simulink library "vhcl2turbLinearize_cl"  (R2020a)
settings: Solver=VariableStepAuto  StartTime=0.0  StopTime=10.0  RelTol=1e-3
undefined symbols (not defined in the file): env, VEHICLE, vhcl
libraries: vrlib x2, addedMass_cl x1, Copy_of_fluidDynamicSurface_cl x1, alphaBeta_ul x1, dragTurbineMantaNew_ul x1, fuselage_cl x1, sixDoFDynamics_cl x1, tethersMoment_cl x1, thrAttachPtKinematics_ul x1
settings Model: Creator=mcobb  LastModifiedBy=andre
settings DataIOCC: ReturnWorkspaceOutputs=off
settings DebuggingCC: ArithmeticOperatorsInVariantConditions=warning
settings SFSimCC: CustomCodeUndefinedFunction=UseInterfaceOnly

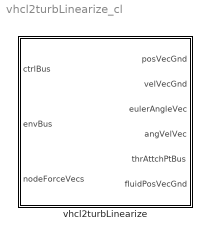
== system vhcl2turbLinearize_cl ==
  vhcl2turbLinearize : Subsystem  VariantControl=strcmpi(VEHICLE,'vehicleManta2Rot')  mask{vcl=vhcl, rho=env.water.density.Value, grav=env.gravAccel.Value}
      mask prompts: vcl "Vehicle"; rho "Density"; grav "Gravity"
      mask DialogControl Container9 Prompt: General
      mask DialogControl Container5 Prompt: Vehicle object (OCT.vehicle)
      mask DialogControl ParameterGroupVar Prompt: Environment Object (OCT.env)
      mask Display:
      | image('kite2.PNG',[0 0 700 700]/4,'on')
      | 
      | port_label('input',1,'ctrlBus')
      | port_label('input',2,'envBus')
      | port_label('input',3,'nodeForceVecs')
      | 
      | port_label('output',1,'posVecGnd')
      | port_label('output',2,'velVecGnd')
      | port_label('output',3,'eulAng')
      | port_label('output',4,'angVelVec')
      | port_label('output',5,'thrAttchPtBus')
      | port_label('output',6,'fluidPosVecGnd')

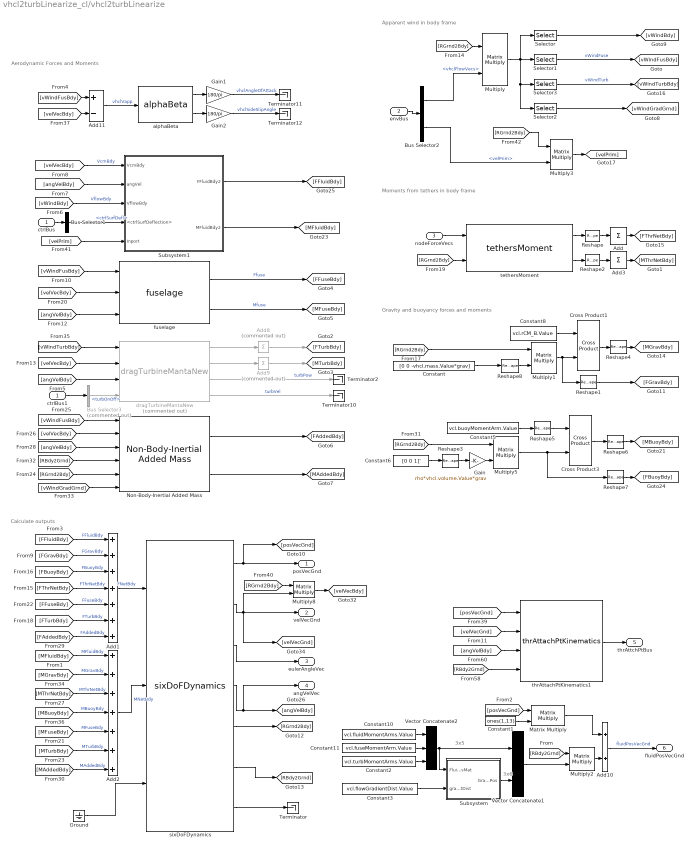
== system vhcl2turbLinearize_cl/vhcl2turbLinearize ==
  note: 3x6
  note: 3x5
  note: Calculate outputs
  note: Apparent wind in body frame
  note: Gravity and buoyancy forces and moments
  note: Moments from tethers in body frame
  note: Aerodynamic Forces and Moments
  ctrlBus : Inport  OutDataTypeStr=Bus: fltCtrlBus
  envBus : Inport  Port=2  OutDataTypeStr=Bus: envBus
  nodeForceVecs : Inport  Port=3
  Add : Sum  Inputs=+  CollapseMode=Specified dimension  CollapseDim=2
  Add1 : Sum  Inputs=+++++++
  Add10 : Sum
  Add11 : Sum  Inputs=+-
  Add2 : Sum  Inputs=+++++++
  Add3 : Sum  Inputs=+  CollapseMode=Specified dimension  CollapseDim=2
  Add8 : Sum  Commented=on  Inputs=1  CollapseMode=Specified dimension  CollapseDim=2
  Add9 : Sum  Commented=on  Inputs=1  CollapseMode=Specified dimension  CollapseDim=2
  Bus Selector1 : BusSelector  OutputSignals=ctrlSurfDefl
  Bus Selector2 : BusSelector  OutputSignals=vhclFlowVecs,velPrim
  Bus Selector3 : BusSelector  Commented=on  OutputSignals=turbOnOff
  Constant : Constant  Value=[0 0 -vhcl.mass.Value*grav]
  Constant1 : Constant  Value=ones(1,13)  VectorParams1D=off
  Constant10 : Constant  Value=vcl.fluidMomentArms.Value
  Constant11 : Constant  Value=vcl.fuseMomentArm.Value
  Constant2 : Constant  Value=vcl.turbMomentArms.Value
  Constant3 : Constant  Value=vcl.flowGradientDist.Value
  Constant5 : Constant  Value=vcl.buoyMomentArm.Value
  Constant6 : Constant  Value=[0 0 1]'
  Constant8 : Constant  Value=vcl.rCM_B.Value
  Cross Product1 : vrlib/Utilities/Cross Product
  Cross Product3 : vrlib/Utilities/Cross Product
  Gain : Gain  Gain=rho*vhcl.volume.Value*grav
  Gain1 : Gain  Gain=180/pi
  Gain2 : Gain  Gain=180/pi
  Ground : Ground
  Matrix Multiply : Product  Multiplication=Matrix(*)
  Multiply{,1..3,5,8} (6 alike) : Product  Multiplication=Matrix(*)
  Non-Body-Inertial Added Mass : addedMass_cl/Non-Body-Inertial Added Mass  MaMat=vcl.Ma6x6_LE.Value  rB_LE=vcl.rB_LE.Value  gradDist=vcl.flowGradientDist.Value
  Reshape : Reshape  OutputDimensionality=Customize  OutputDimensions=[3 vcl.numTethers.Value]
  Reshape{1,3..8} (7 alike) : Reshape  OutputDimensionality=Column vector (2-D)
  Reshape2 : Reshape  OutputDimensionality=Customize  OutputDimensions=[3 vcl.numTethers.Value]
  Selector : Selector  NumberOfDimensions=2  InputPortWidth=3  IndexOptions=Select all,Index vector (dialog)  Indices=[1 3],1:4  OutputSizes=1,1
  Selector1 : Selector  NumberOfDimensions=2  InputPortWidth=3  IndexOptions=Select all,Index vector (dialog)  Indices=[1 3],5  OutputSizes=1,1
  Selector2 : Selector  NumberOfDimensions=2  InputPortWidth=3  IndexOptions=Select all,Index vector (dialog)  Indices=[1 3],8:13  OutputSizes=1,1
  Selector3 : Selector  NumberOfDimensions=2  InputPortWidth=3  IndexOptions=Select all,Index vector (dialog)  Indices=[1 3],6:7  OutputSizes=1,1
  Subsystem : Subsystem
  Subsystem1 : Subsystem
  Terminator{,2,10..12} (5 alike) : Terminator
  Vector Concatenate1 : Concatenate  Mode=Multidimensional array  ConcatenateDimension=2
  Vector Concatenate2 : Concatenate  NumInputs=3  Mode=Multidimensional array  ConcatenateDimension=2
  alphaBeta : alphaBeta_ul/alphaBeta  SystemSampleTime=-1  Latency=0  AutoFrameSizeCalculation=off
  ctrlBus1 : InportShadow  OutDataTypeStr=Bus: fltCtrlBus
  dragTurbineMantaNew : dragTurbineMantaNew_ul/dragTurbineMantaNew  Commented=on  rho_fluid=rho  turb_struct=vcl.struct('OCT.turb')
  fuselage : fuselage_cl/fuselage  momArm=vcl.fuseMomentArm.Value  fus=vcl.fuse  fusRhoDa=rho
  sixDoFDynamics : sixDoFDynamics_cl/sixDoFDynamics  vcl=vcl
      link override sixDoFDynamicsCoupledCM: MMat=vcl.M6x6_B.Value  MaMat=vcl.Ma6x6_LE.Value  rB_LE=vcl.rB_LE.Value
  tethersMoment : tethersMoment_cl/tethersMoment  arms=vcl.struct('OCT.thrAttch')
  thrAttachPtKinematics1 : thrAttachPtKinematics_ul/thrAttachPtKinematics  atchPts=vcl.struct('OCT.thrAttch')
  posVecGnd : Outport  VectorParamsAs1DForOutWhenUnconnected=off
  velVecGnd : Outport  Port=2  VectorParamsAs1DForOutWhenUnconnected=off
  eulerAngleVec : Outport  Port=3  VectorParamsAs1DForOutWhenUnconnected=off
  angVelVec : Outport  Port=4  VectorParamsAs1DForOutWhenUnconnected=off
  thrAttchPtBus : Outport  Port=5  VectorParamsAs1DForOutWhenUnconnected=off
  fluidPosVecGnd : Outport  Port=6  VectorParamsAs1DForOutWhenUnconnected=off
  wires:
  sixDoFDynamics/3 -> eulerAngleVec/1
  sixDoFDynamics/1 -> [posVecGnd], posVecGnd/1
  sixDoFDynamics/2 -> Multiply8/2, [velVecGnd], velVecGnd/1
  thrAttachPtKinematics1/1 -> thrAttchPtBus/1
  ctrlBus/1 -> Bus Selector1/1
  [vWindFusBdy] -> fuselage/1
  [velVecBdy] -> fuselage/2
  [angVelBdy] -> fuselage/3
  [vWindTurbBdy] -> dragTurbineMantaNew/1
  [velVecBdy] -> dragTurbineMantaNew/2
  [angVelBdy] -> dragTurbineMantaNew/3
  dragTurbineMantaNew/1 -> Add8/1
  dragTurbineMantaNew/2 -> Add9/1
  Add8/1 -> [FTurbBdy]
  Add9/1 -> [MTurbBdy]
  dragTurbineMantaNew/3 -> Terminator2/1  "turbPow"
  [vWindFusBdy] -> Non-Body-Inertial Added Mass/1
  [velVecBdy] -> Non-Body-Inertial Added Mass/2
  [angVelBdy] -> Non-Body-Inertial Added Mass/3
  [RBdy2Grnd] -> Non-Body-Inertial Added Mass/4
  [RGrnd2Bdy] -> Non-Body-Inertial Added Mass/5
  [vWindGradGrnd] -> Non-Body-Inertial Added Mass/6
  Constant6/1 -> Reshape3/1
  Reshape3/1 -> Gain/1
  [RGrnd2Bdy] -> Multiply5/1
  Gain/1 -> Multiply5/2
  Constant5/1 -> Reshape5/1
  Reshape5/1 -> Cross Product3/1
  Cross Product3/1 -> Reshape6/1
  Reshape6/1 -> [MBuoyBdy]
  Multiply5/1 -> Reshape7/1, Cross Product3/2
  Reshape7/1 -> [FBuoyBdy]
  Reshape1/1 -> [FGravBdy]
  Multiply1/1 -> Reshape1/1, Cross Product1/2
  fuselage/1 -> [FFuseBdy]  "Ffuse"
  fuselage/2 -> [MFuseBdy]  "Mfuse"
  Constant/1 -> Reshape8/1
  [RGrnd2Bdy] -> Multiply1/1
  Reshape8/1 -> Multiply1/2
  Constant8/1 -> Cross Product1/1
  Cross Product1/1 -> Reshape4/1
  Reshape4/1 -> [MGravBdy]
  [RGrnd2Bdy] -> tethersMoment/2
  nodeForceVecs/1 -> tethersMoment/1
  tethersMoment/1 -> Reshape/1
  tethersMoment/2 -> Reshape2/1
  Reshape/1 -> Add/1
  Reshape2/1 -> Add3/1
  Add/1 -> [FThrNetBdy]
  Add3/1 -> [MThrNetBdy]
  [RGrnd2Bdy] -> Multiply/1
  envBus/1 -> Bus Selector2/1
  Bus Selector2/1 -> Multiply/2  "<vhclFlowVecs>"
  Multiply/1 -> Selector/1, Selector2/1, Selector3/1, Selector1/1
  Selector/1 -> [vWindBdy]
  Selector1/1 -> [vWindFusBdy]  "vWindFuse"
  Selector2/1 -> [vWindGradGrnd]
  [RGrnd2Bdy] -> Multiply8/1
  Multiply8/1 -> [velVecBdy]
  [FFluidBdy] -> Add1/1  "FFluidBdy"
  [FGravBdy] -> Add1/2  "FGravBdy"
  [FBuoyBdy] -> Add1/3  "FBuoyBdy"
  [FThrNetBdy] -> Add1/4  "FThrNetBdy"
  [FFuseBdy] -> Add1/5  "FFuseBdy"
  [FTurbBdy] -> Add1/6  "FTurbBdy"
  [FAddedBdy] -> Add1/7  "FAddedBdy"
  Add1/1 -> sixDoFDynamics/1  "FNetBdy"
  [MFluidBdy] -> Add2/1  "MFluidBdy"
  [MGravBdy] -> Add2/2  "MGravBdy"
  [MThrNetBdy] -> Add2/3  "MThrNetBdy"
  [MBuoyBdy] -> Add2/4  "MBuoyBdy"
  [MFuseBdy] -> Add2/5  "MFuseBdy"
  [MTurbBdy] -> Add2/6  "MTurbBdy"
  [MAddedBdy] -> Add2/7  "MAddedBdy"
  Add2/1 -> sixDoFDynamics/2  "MNetBdy"
  sixDoFDynamics/5 -> [RGrnd2Bdy]
  sixDoFDynamics/6 -> [RBdy2Grnd]
  [posVecGnd] -> thrAttachPtKinematics1/1
  [velVecGnd] -> thrAttachPtKinematics1/2
  [angVelBdy] -> thrAttachPtKinematics1/3
  [RBdy2Grnd] -> thrAttachPtKinematics1/4
  Constant10/1 -> Vector Concatenate2/1
  Constant11/1 -> Vector Concatenate2/2
  Vector Concatenate2/1 -> Vector Concatenate1/1, Subsystem/1(FluidCentPosMat)
  Constant3/1 -> Subsystem/2(gradientDist)
  Subsystem/1(GradientFlowPos) -> Vector Concatenate1/2
  sixDoFDynamics/4 -> [angVelBdy], angVelVec/1
  Vector Concatenate1/1 -> Multiply2/2
  [RBdy2Grnd] -> Multiply2/1
  Multiply2/1 -> Add10/2
  Matrix Multiply/1 -> Add10/1
  Add10/1 -> fluidPosVecGnd/1  "fluidPosVecGnd"
  Constant1/1 -> Matrix Multiply/2
  [posVecGnd] -> Matrix Multiply/1
  Bus Selector3/1 -> dragTurbineMantaNew/4  "<turbOnOff>"
  ctrlBus1/1 -> Bus Selector3/1
  Constant2/1 -> Vector Concatenate2/3
  Selector3/1 -> [vWindTurbBdy]  "vWindTurb"
  dragTurbineMantaNew/4 -> Terminator10/1  "turbVel"
  Non-Body-Inertial Added Mass/1 -> [FAddedBdy]
  Non-Body-Inertial Added Mass/2 -> [MAddedBdy]
  [vWindFusBdy] -> Add11/1
  Add11/1 -> alphaBeta/1  "vhclVapp"
  [velVecBdy] -> Add11/2
  alphaBeta/2 -> Gain2/1
  Gain1/1 -> Terminator11/1  "vhclAngleOfAttack"
  alphaBeta/1 -> Gain1/1
  Gain2/1 -> Terminator12/1  "vhclSideSlipAngle"
  [velVecBdy] -> Subsystem1/1(VcmBdy)  "VcmBdy"
  [angVelBdy] -> Subsystem1/2(angVel)
  [vWindBdy] -> Subsystem1/3(VflowBdy)  "VflowBdy"
  Bus Selector1/1 -> Subsystem1/4(<ctrlSurfDeflection>)  "<ctrlSurfDefl>"
  Subsystem1/1(FFluidBdy2) -> [FFluidBdy]
  Subsystem1/2(MFluidBdy2) -> [MFluidBdy]
  Bus Selector2/2 -> Multiply3/2  "<velPrim>"
  [velPrim] -> Subsystem1/5(Inport)
  [RGrnd2Bdy] -> Multiply3/1
  Multiply3/1 -> [velPrim]
  Ground/1 -> sixDoFDynamics/3
  sixDoFDynamics/7 -> Terminator/1

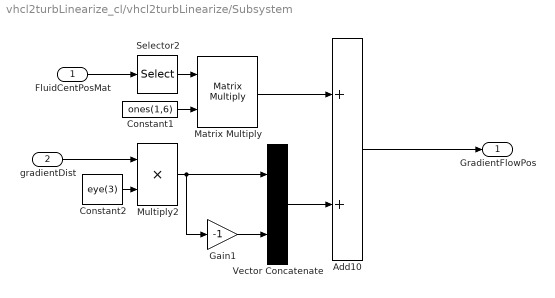
== system vhcl2turbLinearize_cl/vhcl2turbLinearize/Subsystem ==
  FluidCentPosMat : Inport
  gradientDist : Inport  Port=2
  Add10 : Sum
  Constant1 : Constant  Value=ones(1,6)  VectorParams1D=off
  Constant2 : Constant  Value=eye(3)
  Gain1 : Gain  Gain=-1
  Matrix Multiply : Product  Multiplication=Matrix(*)
  Multiply2 : Product
  Selector2 : Selector  NumberOfDimensions=2  InputPortWidth=3  IndexOptions=Select all,Index vector (dialog)  Indices=[1 3],5  OutputSizes=1,1
  Vector Concatenate : Concatenate  Mode=Multidimensional array  ConcatenateDimension=2
  GradientFlowPos : Outport  VectorParamsAs1DForOutWhenUnconnected=off
  wires:
  FluidCentPosMat/1 -> Selector2/1
  Vector Concatenate/1 -> Add10/2
  Selector2/1 -> Matrix Multiply/1
  Multiply2/1 -> Gain1/1, Vector Concatenate/1
  Constant1/1 -> Matrix Multiply/2
  Matrix Multiply/1 -> Add10/1
  Gain1/1 -> Vector Concatenate/2
  Constant2/1 -> Multiply2/2
  Add10/1 -> GradientFlowPos/1
  gradientDist/1 -> Multiply2/1

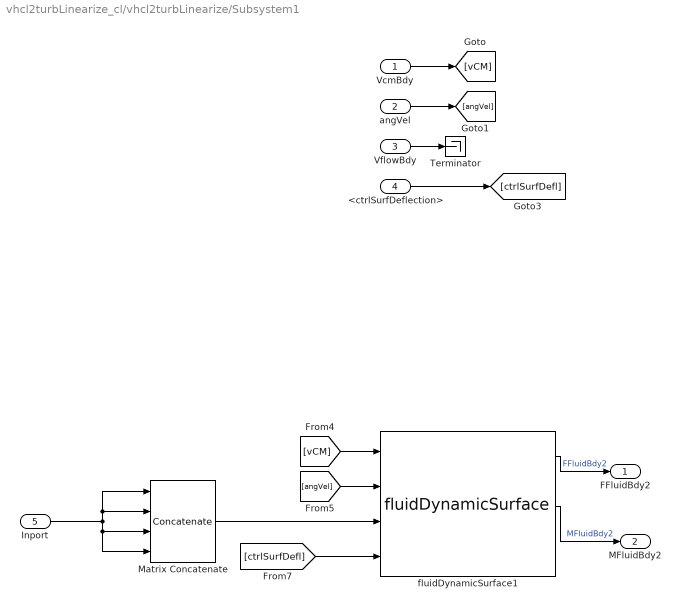
== system vhcl2turbLinearize_cl/vhcl2turbLinearize/Subsystem1 ==
  VcmBdy : Inport
  angVel : Inport  Port=2
  VflowBdy : Inport  Port=3
  <ctrlSurfDeflection> : Inport  Port=4
  Inport : Inport  Port=5
  Matrix Concatenate : Concatenate  NumInputs=4  Mode=Multidimensional array  ConcatenateDimension=2
  Terminator : Terminator
  fluidDynamicSurface1 : Copy_of_fluidDynamicSurface_cl/fluidDynamicSurface  vcl=vcl  fluidDensity=env.water.density.Value  fluidMomentArms=vcl.fluidMomentArms.Value  fluidRefArea=vcl.fluidRefArea.Value  wingTips=vcl.wingTipPositions.Value
  FFluidBdy2 : Outport
  MFluidBdy2 : Outport  Port=2
  wires:
  angVel/1 -> [angVel]
  <ctrlSurfDeflection>/1 -> [ctrlSurfDefl]
  VflowBdy/1 -> Terminator/1
  VcmBdy/1 -> [vCM]
  Inport/1 -> Matrix Concatenate/4, Matrix Concatenate/3, Matrix Concatenate/2, Matrix Concatenate/1
  [angVel] -> fluidDynamicSurface1/2
  [vCM] -> fluidDynamicSurface1/1
  [ctrlSurfDefl] -> fluidDynamicSurface1/4
  fluidDynamicSurface1/1 -> FFluidBdy2/1  "FFluidBdy2"
  fluidDynamicSurface1/2 -> MFluidBdy2/1  "MFluidBdy2"
  Matrix Concatenate/1 -> fluidDynamicSurface1/3
